simulink model "StraightWithLeadingCar_cs"  (R2016a)
settings: Solver=ode5  SolverMode=SingleTasking  StartTime=0.0  StopTime=40  FixedStep=1/1000  RelTol=1e-3
PreLoadFcn:
  | mbxruntime.callbacks.PreLoadFcn(bdroot);
PostLoadFcn:
  | mbxruntime.callbacks.PostLoadFcn(bdroot);
InitFcn:
  | mbxruntime.callbacks.InitFcn(bdroot);
StartFcn:
  | mbxruntime.callbacks.StartFcn(bdroot);
StopFcn:
  | mbxruntime.callbacks.StopFcn(bdroot);
model workspace (MAT data in the model file):
  mbox_table : struct (value not decoded)
  model_closed = 0
  sim_status = 0
values from neighbouring files (symbols this model uses):
  ACCDuration = 5    [PreScan_Runscript.m]
  V0 = ACCArray(2*ACCCasei-1)    [PreScan_Runscript.m]
  V1 = ACCArray(2*ACCCasei)    [PreScan_Runscript.m]
  VAccuracyIn = 0.8    [PreScan_Runscript.m]
  VDurationIn = 2    [PreScan_Runscript.m]
  VPIDIn = ACCArray(2*ACCCasei-1)    [PreScan_Runscript.m]
  VToleranceIn = 1    [PreScan_Runscript.m]
undefined symbols (not defined in the file or in its folder): ADASID, BMotor1, BMotor2, BrkDelayTime, DControlB, Delay1, Delay2, DiscIntNeverNeededParam, IControlB, JMotor1, JMotor2, mbxruntime, PControlB, PreScanCarSimLoadFcn, ratioGearF, ratioGearR, tabledata, TorqDelayTime, Tstep
undefined symbols (not defined in the file): SteeringColumn, SteeringWheel, WheelL0, WheelL1, WheelR0, WheelR1
libraries: simulink x14, simulink_extras x11, PreScanSimulinkLibrary x9, MyLib x3, Solver_SF x2, PreScanUsefulBlocks x2, pil_lib x1
(part 9 of 12)

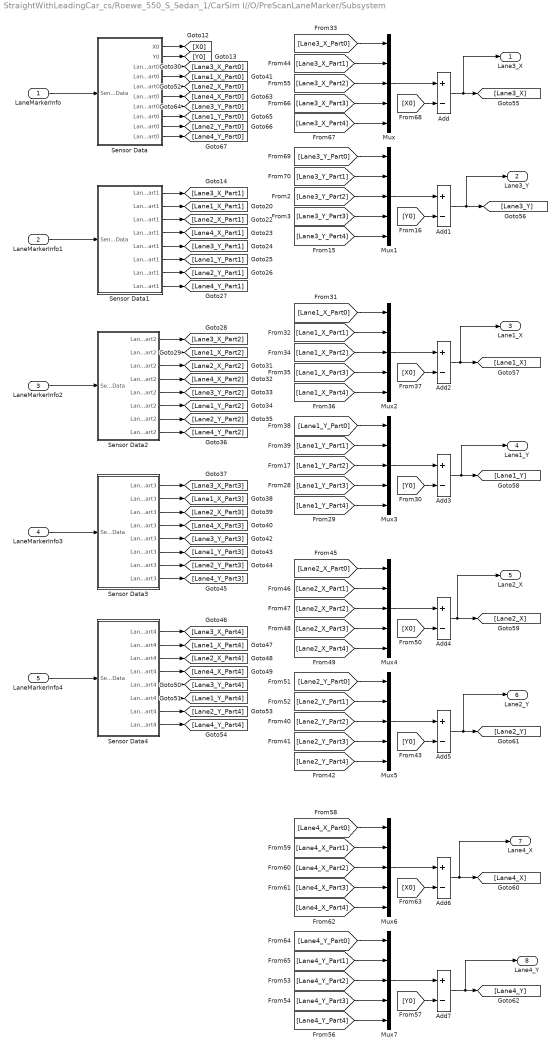
== system StraightWithLeadingCar_cs/Roewe_550_S_Sedan_1/CarSim I//O/PreScanLaneMarker/Subsystem ==
  LaneMarkerInfo : Inport
  LaneMarkerInfo1 : Inport  Port=2
  LaneMarkerInfo2 : Inport  Port=3
  LaneMarkerInfo3 : Inport  Port=4
  LaneMarkerInfo4 : Inport  Port=5
  Add{,1..7} (8 alike) : Sum  Inputs=+-
  Mux{,1..7} (8 alike) : Mux  Inputs=5
  Sensor Data : Subsystem
  Sensor Data1 : Subsystem
  Sensor Data2 : Subsystem
  Sensor Data3 : Subsystem
  Sensor Data4 : Subsystem
  Lane3_X : Outport
  Lane3_Y : Outport  Port=2
  Lane1_X : Outport  Port=3
  Lane1_Y : Outport  Port=4
  Lane2_X : Outport  Port=5
  Lane2_Y : Outport  Port=6
  Lane4_X : Outport  Port=7
  Lane4_Y : Outport  Port=8
  wires:
  [X0] -> Add4/2
  [Lane4_X_Part2] -> Mux6/3
  [Lane2_Y_Part1] -> Mux5/2
  Mux6/1 -> Add6/1
  [Lane4_X_Part0] -> Mux6/1
  [X0] -> Add6/2
  [Lane4_Y_Part4] -> Mux7/5
  Add/1 -> Lane3_X/1, [Lane3_X]
  [Lane4_Y_Part0] -> Mux7/1
  Add3/1 -> Lane1_Y/1, [Lane1_Y]
  [Lane2_Y_Part0] -> Mux5/1
  Mux5/1 -> Add5/1
  Add6/1 -> Lane4_X/1, [Lane4_X]
  [Lane2_Y_Part3] -> Mux5/4
  Mux7/1 -> Add7/1
  Add4/1 -> Lane2_X/1, [Lane2_X]
  Add1/1 -> Lane3_Y/1, [Lane3_Y]
  [Y0] -> Add5/2
  [Lane4_Y_Part1] -> Mux7/2
  [Lane2_Y_Part2] -> Mux5/3
  [Lane4_Y_Part2] -> Mux7/3
  [Lane4_X_Part3] -> Mux6/4
  [Lane4_X_Part4] -> Mux6/5
  [Y0] -> Add7/2
  [Lane4_X_Part1] -> Mux6/2
  Add7/1 -> Lane4_Y/1, [Lane4_Y]
  Add5/1 -> Lane2_Y/1, [Lane2_Y]
  [Lane4_Y_Part3] -> Mux7/4
  [Lane2_Y_Part4] -> Mux5/5
  Sensor Data4/5(Lane3_Y_Part4) -> [Lane3_Y_Part4]
  Sensor Data2/7(Lane2_Y_Part2) -> [Lane2_Y_Part2]
  Sensor Data3/5(Lane3_Y_Part3) -> [Lane3_Y_Part3]
  [Lane3_X_Part3] -> Mux/4
  Sensor Data2/1(Lane3_X_Part2) -> [Lane3_X_Part2]
  Sensor Data3/1(Lane3_X_Part3) -> [Lane3_X_Part3]
  Sensor Data1/8(Lane4_Y_Part1) -> [Lane4_Y_Part1]
  Sensor Data3/3(Lane2_X_Part3) -> [Lane2_X_Part3]
  Sensor Data4/3(Lane2_X_Part4) -> [Lane2_X_Part4]
  Sensor Data2/6(Lane1_Y_Part2) -> [Lane1_Y_Part2]
  Sensor Data1/6(Lane1_Y_Part1) -> [Lane1_Y_Part1]
  Sensor Data3/2(Lane1_X_Part3) -> [Lane1_X_Part3]
  Sensor Data2/3(Lane2_X_Part2) -> [Lane2_X_Part2]
  Sensor Data3/8(Lane4_Y_Part3) -> [Lane4_Y_Part3]
  Sensor Data4/2(Lane1_X_Part4) -> [Lane1_X_Part4]
  Sensor Data3/7(Lane2_Y_Part3) -> [Lane2_Y_Part3]
  Sensor Data4/7(Lane2_Y_Part4) -> [Lane2_Y_Part4]
  Sensor Data3/6(Lane1_Y_Part3) -> [Lane1_Y_Part3]
  [Lane3_X_Part4] -> Mux/5
  [Lane3_X_Part1] -> Mux/2
  Sensor Data4/4(Lane4_X_Part4) -> [Lane4_X_Part4]
  [X0] -> Add/2
  Sensor Data2/2(Lane1_X_Part2) -> [Lane1_X_Part2]
  Sensor Data1/3(Lane2_X_Part1) -> [Lane2_X_Part1]
  Sensor Data4/6(Lane1_Y_Part4) -> [Lane1_Y_Part4]
  [Lane3_X_Part0] -> Mux/1
  Mux/1 -> Add/1
  [Lane3_Y_Part0] -> Mux1/1
  [Lane3_Y_Part2] -> Mux1/3
  [Lane3_Y_Part4] -> Mux1/5
  [Lane3_Y_Part1] -> Mux1/2
  Mux1/1 -> Add1/1
  [Y0] -> Add1/2
  Sensor Data2/8(Lane4_Y_Part2) -> [Lane4_Y_Part2]
  [Lane1_X_Part4] -> Mux2/5
  [Lane1_Y_Part0] -> Mux3/1
  [Lane1_X_Part3] -> Mux2/4
  [Lane1_Y_Part3] -> Mux3/4
  Sensor Data2/5(Lane3_Y_Part2) -> [Lane3_Y_Part2]
  Sensor Data1/7(Lane2_Y_Part1) -> [Lane2_Y_Part1]
  Sensor Data4/1(Lane3_X_Part4) -> [Lane3_X_Part4]
  Sensor Data4/8(Lane4_Y_Part4) -> [Lane4_Y_Part4]
  Sensor Data3/4(Lane4_X_Part3) -> [Lane4_X_Part3]
  Sensor Data2/4(Lane4_X_Part2) -> [Lane4_X_Part2]
  [Lane3_Y_Part3] -> Mux1/4
  Sensor Data1/5(Lane3_Y_Part1) -> [Lane3_Y_Part1]
  [Lane1_X_Part1] -> Mux2/2
  [Lane1_X_Part2] -> Mux2/3
  Mux2/1 -> Add2/1
  [X0] -> Add2/2
  [Lane1_X_Part0] -> Mux2/1
  [Lane1_Y_Part2] -> Mux3/3
  [Lane1_Y_Part4] -> Mux3/5
  [Lane3_X_Part2] -> Mux/3
  [Y0] -> Add3/2
  [Lane2_X_Part0] -> Mux4/1
  [Lane2_X_Part2] -> Mux4/3
  [Lane1_Y_Part1] -> Mux3/2
  Mux3/1 -> Add3/1
  Mux4/1 -> Add4/1
  [Lane2_X_Part3] -> Mux4/4
  [Lane2_X_Part1] -> Mux4/2
  [Lane2_X_Part4] -> Mux4/5
  Sensor Data/2(Y0) -> [Y0]
  Sensor Data/3(Lane3_X_Part0) -> [Lane3_X_Part0]
  Sensor Data/6(Lane4_X_Part0) -> [Lane4_X_Part0]
  Sensor Data/7(Lane3_Y_Part0) -> [Lane3_Y_Part0]
  Sensor Data/1(X0) -> [X0]
  Sensor Data/4(Lane1_X_Part0) -> [Lane1_X_Part0]
  Sensor Data/8(Lane1_Y_Part0) -> [Lane1_Y_Part0]
  Sensor Data/9(Lane2_Y_Part0) -> [Lane2_Y_Part0]
  Sensor Data/10(Lane4_Y_Part0) -> [Lane4_Y_Part0]
  Sensor Data1/1(Lane3_X_Part1) -> [Lane3_X_Part1]
  Sensor Data/5(Lane2_X_Part0) -> [Lane2_X_Part0]
  Sensor Data1/2(Lane1_X_Part1) -> [Lane1_X_Part1]
  Sensor Data1/4(Lane4_X_Part1) -> [Lane4_X_Part1]
  Add2/1 -> Lane1_X/1, [Lane1_X]
  LaneMarkerInfo/1 -> Sensor Data/1(Sensor Data)
  LaneMarkerInfo1/1 -> Sensor Data1/1(Sensor Data)
  LaneMarkerInfo2/1 -> Sensor Data2/1(Sensor Data)
  LaneMarkerInfo3/1 -> Sensor Data3/1(Sensor Data)
  LaneMarkerInfo4/1 -> Sensor Data4/1(Sensor Data)

== system StraightWithLeadingCar_cs/Roewe_550_S_Sedan_1/CarSim_Vehicle/CarSim2PreScanSTATE/Transformation_SprungMassCarSim2PreScan ==
  In1 : Inport
  Demux : Demux  Outputs=3
  Ini z-position VEHICLE wrt GLOBAL axis system [m] : Constant  Value=z0
  Mux : Mux  Inputs=3
  Sum1 : Sum  Inputs=+-
  Out1 : Outport
  wires:
  Mux/1 -> Out1/1
  Ini z-position VEHICLE wrt GLOBAL axis system [m]/1 -> Sum1/2
  Demux/1 -> Mux/1
  Sum1/1 -> Mux/3
  Demux/3 -> Sum1/1
  Demux/2 -> Mux/2
  In1/1 -> Demux/1

== system StraightWithLeadingCar_cs/Roewe_550_S_Sedan_1/CarSim_Vehicle/CarSim2PreScan_BUS/Steering ==
  SteeringWheel_In : Inport
  AvoidDivisionByZero : Subsystem
  Bus Creator4 : BusCreator  Inputs=1
  DefaultValue : Constant  Value=16
  Demux2 : Demux  Outputs=2
  Divide : Product  Inputs=*/
  Switch : Switch  Criteria=u2 ~= 0
  Steering : Outport
  wires:
  AvoidDivisionByZero/1(Out1) -> Divide/2
  Switch/1 -> Bus Creator4/1  "SteeringRatio_[-]"
  DefaultValue/1 -> Switch/3
  Divide/1 -> Switch/1, Switch/2  "Steering_Ration[-]"
  Demux2/2 -> AvoidDivisionByZero/1(In1)  "Axle1ReducedSW"
  Demux2/1 -> Divide/1  "SteeringWheelAngle_[deg]"
  Bus Creator4/1 -> Steering/1  "Steering"
  SteeringWheel_In/1 -> Demux2/1

== system StraightWithLeadingCar_cs/Roewe_550_S_Sedan_1/CarSim_Vehicle/CarSim2PreScan_BUS/Vehicle ==
  v_VehicleCoG[x;y;z][km|h] : Inport
  Bus Creator1 : BusCreator  Inputs=1
  Bus Creator7 : BusCreator  Inputs=1
  Bus Creator8 : BusCreator  Inputs=3
  Demux : Demux  Outputs=3
  Vehicle : Outport
  wires:
  Demux/3 -> Bus Creator8/3  "v_Vehicle[z][km|h]"
  Demux/2 -> Bus Creator8/2  "v_Vehicle[y][km|h]"
  Demux/1 -> Bus Creator8/1  "v_Vehicle[x][km|h]"
  Bus Creator7/1 -> Bus Creator1/1  "Velocities"
  Bus Creator8/1 -> Bus Creator7/1  "Linear"
  Bus Creator1/1 -> Vehicle/1  "Vehicle"
  v_VehicleCoG[x;y;z][km|h]/1 -> Demux/1

== system StraightWithLeadingCar_cs/Roewe_550_S_Sedan_1/CarSim_Vehicle/CarSim2PreScan_BUS/Wheel ==
  SprungMass_Pos_Global[x;y;z][m] : Inport
  SprungMass_Angle_Global[x;y;z][deg] : Inport  Port=2
  CarSim_Pos_Wheel_[FL;FR;RL;RR][x;y;z][m] : Inport  Port=3
  CarSim_Angle_Wheel_[FL;FR;RL;RR][x;y;z][deg;rev;deg] : Inport  Port=4
  Bus Creator3 : BusCreator  Inputs=2
  Bus Creator6 : BusCreator  Inputs=1
  Convert CarSim to PreScan Wheel Position : Subsystem
  Convert CarSim to PreScan Wheel Rotation : Subsystem
  Demux : Demux  Outputs=[3 3 3 3]
  Demux1 : Demux  Outputs=[3 3 3 3]
  Wheel : Outport
  wires:
  SprungMass_Angle_Global[x;y;z][deg]/1 -> Convert CarSim to PreScan Wheel Rotation/5(Angle_Vehicle[x;y;z][deg]), Convert CarSim to PreScan Wheel Position/2(SprungMass_Angle_Global[x;y;z][deg])
  SprungMass_Pos_Global[x;y;z][m]/1 -> Convert CarSim to PreScan Wheel Position/1(SprungMass_Pos_Global[x;y;z][m])
  CarSim_Angle_Wheel_[FL;FR;RL;RR][x;y;z][deg;rev;deg]/1 -> Demux1/1
  Demux1/4 -> Convert CarSim to PreScan Wheel Rotation/4(CarSim_Angle_RR_Wheel_CoorSys_V[deg;rev;deg])  "CarSim_Angle_RR_Wheel_CoorSys_V[deg;rev;deg]"
  Demux1/3 -> Convert CarSim to PreScan Wheel Rotation/3(CarSim_Angle_RL_Wheel_CoorSys_V[deg;rev;deg])  "CarSim_Angle_RL_Wheel_CoorSys_V[deg;rev;deg]"
  Demux1/2 -> Convert CarSim to PreScan Wheel Rotation/2(CarSim_Angle_FR_Wheel_CoorSys_V[deg;rev;deg])  "CarSim_Angle_FR_Wheel_CoorSys_V[deg;rev;deg]"
  Demux1/1 -> Convert CarSim to PreScan Wheel Rotation/1(CarSim_Angle_FL_Wheel_CoorSys_V[deg;rev;deg])  "CarSim_Angle_FL_Wheel_CoorSys_V[deg;rev;deg]"
  CarSim_Pos_Wheel_[FL;FR;RL;RR][x;y;z][m]/1 -> Demux/1
  Demux/4 -> Convert CarSim to PreScan Wheel Position/6(CarSim_Pos_RR_Wheel[x;y;z][m])  "CarSim_Pos_RR_Wheel[x;y;z][m]"
  Demux/3 -> Convert CarSim to PreScan Wheel Position/5(CarSim_Pos_RL_Wheel[x;y;z][m])  "CarSim_Pos_RL_Wheel[x;y;z][m]"
  Demux/2 -> Convert CarSim to PreScan Wheel Position/4(CarSim_Pos_FR_Wheel[x;y;z][m])  "CarSim_Pos_FR_Wheel[x;y;z][m]"
  Demux/1 -> Convert CarSim to PreScan Wheel Position/3(CarSim_Pos_FL_Wheel[x;y;z][m])  "CarSim_Pos_FL_Wheel[x;y;z][m]"
  Bus Creator6/1 -> Wheel/1  "Wheel"
  Bus Creator3/1 -> Bus Creator6/1  "Position"
  Convert CarSim to PreScan Wheel Rotation/1(PreScanWheel_Rot) -> Bus Creator3/2
  Convert CarSim to PreScan Wheel Position/1(PreScanWheel_Pos) -> Bus Creator3/1

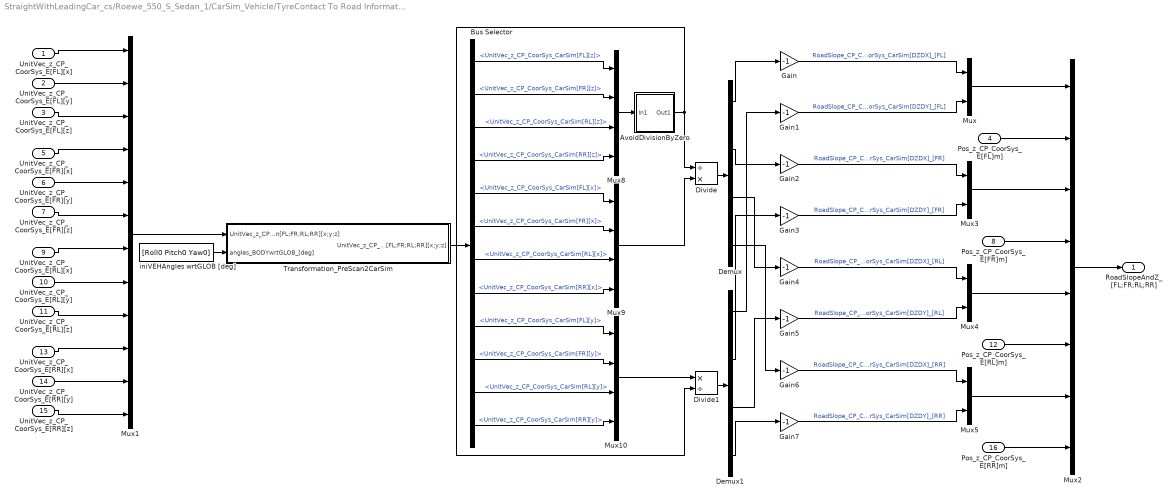
== system StraightWithLeadingCar_cs/Roewe_550_S_Sedan_1/CarSim_Vehicle/TyreContact To Road Information/Contact To Road Information ==
  UnitVec_z_CP_CoorSys_E[FL][x] : Inport
  UnitVec_z_CP_CoorSys_E[FL][y] : Inport  Port=2
  UnitVec_z_CP_CoorSys_E[FL][z] : Inport  Port=3
  " Pos_z_CP_CoorSys_E[FL]m]" : Inport  Port=4
  UnitVec_z_CP_CoorSys_E[FR][x] : Inport  Port=5
  UnitVec_z_CP_CoorSys_E[FR][y] : Inport  Port=6
  UnitVec_z_CP_CoorSys_E[FR][z] : Inport  Port=7
  " Pos_z_CP_CoorSys_E[FR]m]" : Inport  Port=8
  UnitVec_z_CP_CoorSys_E[RL][x] : Inport  Port=9
  UnitVec_z_CP_CoorSys_E[RL][y] : Inport  Port=10
  UnitVec_z_CP_CoorSys_E[RL][z] : Inport  Port=11
  " Pos_z_CP_CoorSys_E[RL]m]" : Inport  Port=12
  UnitVec_z_CP_CoorSys_E[RR][x] : Inport  Port=13
  UnitVec_z_CP_CoorSys_E[RR][y] : Inport  Port=14
  UnitVec_z_CP_CoorSys_E[RR][z] : Inport  Port=15
  " Pos_z_CP_CoorSys_E[RR]m]" : Inport  Port=16
  AvoidDivisionByZero : Subsystem
  Bus Selector : BusSelector  OutputSignals=UnitVec_z_CP_CoorSys_CarSim[FL][x;y;z].UnitVec_z_CP_CoorSys_CarSim[FL][z],UnitVec_z_CP_CoorSys_CarSim[FR][x;y;z].UnitVec_z_CP_CoorSys_CarSim[FR][z],UnitVec_z_CP_CoorSys_CarSim[RL][x;y;z].UnitVec_z_CP_CoorSys_CarSim[RL][z],UnitVec_z_CP_CoorSys_CarSim[RR][x;y;z].UnitVec_z_CP_CoorSys_CarSim[RR][z],UnitVec_z_CP_CoorSys_CarSim[FL][x;y;z].UnitVec_z_CP_CoorSys_CarSim[FL][x],UnitVec_z_CP_CoorSys_CarSim[FR][x;y;z].UnitVec_z_CP_CoorSys_CarSim[FR][x],UnitVec_z_CP_CoorSys_CarSim[RL][x;y;z].UnitVec_z_CP_CoorSys_CarSim[RL][x],UnitVec_z_CP_CoorSys_CarSim[RR][x;y;z].UnitVec_z_CP_CoorSys_CarSim[RR][x],UnitVec_z_CP_CoorSys_CarSim[FL][x;y;z].UnitVec_z_CP_CoorSys_CarSim[FL][y],UnitVec_z_CP_CoorSys_CarSim[FR][x;y;z].UnitVec_z_CP_CoorSys_CarSim[FR][y],UnitVec_z_CP_CoorSys_CarSim[RL][x;y;z].UnitVec_z_CP_CoorSys_CarSim[RL][y],UnitVec_z_CP_CoorSys_CarSim[RR][x;y;z].UnitVec_z_CP_CoorSys_CarSim[RR][y]
  Demux : Demux
  Demux1 : Demux
  Divide : Product  Inputs=/*
  Divide1 : Product  Inputs=*/
  Gain{,1..7} (8 alike) : Gain  Gain=-1
  Mux{,3..5} (4 alike) : Mux  Inputs=2
  Mux1 : Mux  Inputs=12
  Mux10 : Mux
  Mux2 : Mux  Inputs=[2 1 2 1 2 1 2 1]
  Mux8 : Mux
  Mux9 : Mux
  Transformation_PreScan2CarSim : Subsystem
  iniVEHAngles wrtGLOB [deg] : Constant  Value=[Roll0 Pitch0 Yaw0]
  RoadSlopeAndZ_[FL;FR;RL;RR] : Outport
  wires:
  AvoidDivisionByZero/1(Out1) -> Divide1/2, Divide/1
  Demux1/4 -> Gain7/1
  Demux/4 -> Gain6/1
  Demux1/3 -> Gain5/1
  Demux/3 -> Gain4/1
  Demux1/2 -> Gain3/1
  Demux/2 -> Gain2/1
  Demux/1 -> Gain/1
  Demux1/1 -> Gain1/1
  Divide1/1 -> Demux1/1
  Divide/1 -> Demux/1
  Mux10/1 -> Divide1/1
  Mux9/1 -> Divide/2
  Mux8/1 -> AvoidDivisionByZero/1(In1)
  Bus Selector/12 -> Mux10/4  "<UnitVec_z_CP_CoorSys_CarSim[RR][y]>"
  Bus Selector/11 -> Mux10/3  "<UnitVec_z_CP_CoorSys_CarSim[RL][y]>"
  Bus Selector/10 -> Mux10/2  "<UnitVec_z_CP_CoorSys_CarSim[FR][y]>"
  Bus Selector/9 -> Mux10/1  "<UnitVec_z_CP_CoorSys_CarSim[FL][y]>"
  Bus Selector/8 -> Mux9/4  "<UnitVec_z_CP_CoorSys_CarSim[RR][x]>"
  Bus Selector/7 -> Mux9/3  "<UnitVec_z_CP_CoorSys_CarSim[RL][x]>"
  Bus Selector/6 -> Mux9/2  "<UnitVec_z_CP_CoorSys_CarSim[FR][x]>"
  Bus Selector/5 -> Mux9/1  "<UnitVec_z_CP_CoorSys_CarSim[FL][x]>"
  Bus Selector/4 -> Mux8/4  "<UnitVec_z_CP_CoorSys_CarSim[RR][z]>"
  Bus Selector/3 -> Mux8/3  "<UnitVec_z_CP_CoorSys_CarSim[RL][z]>"
  Bus Selector/2 -> Mux8/2  "<UnitVec_z_CP_CoorSys_CarSim[FR][z]>"
  Bus Selector/1 -> Mux8/1  "<UnitVec_z_CP_CoorSys_CarSim[FL][z]>"
  Mux5/1 -> Mux2/7
  Mux4/1 -> Mux2/5
  Mux3/1 -> Mux2/3
  " Pos_z_CP_CoorSys_E[FL]m]"/1 -> Mux2/2
  Mux/1 -> Mux2/1
  Gain/1 -> Mux/1  "RoadSlope_CP_CoorSys_CarSim[DZDX]_[FL]"
  " Pos_z_CP_CoorSys_E[RR]m]"/1 -> Mux2/8
  " Pos_z_CP_CoorSys_E[RL]m]"/1 -> Mux2/6
  " Pos_z_CP_CoorSys_E[FR]m]"/1 -> Mux2/4
  Transformation_PreScan2CarSim/1(UnitVec_z_CP_CoorSys _CarSim[FL;FR;RL;RR][x;y;z]) -> Bus Selector/1
  UnitVec_z_CP_CoorSys_E[RR][z]/1 -> Mux1/12
  UnitVec_z_CP_CoorSys_E[RR][y]/1 -> Mux1/11
  UnitVec_z_CP_CoorSys_E[RR][x]/1 -> Mux1/10
  UnitVec_z_CP_CoorSys_E[RL][z]/1 -> Mux1/9
  UnitVec_z_CP_CoorSys_E[RL][y]/1 -> Mux1/8
  UnitVec_z_CP_CoorSys_E[RL][x]/1 -> Mux1/7
  UnitVec_z_CP_CoorSys_E[FR][z]/1 -> Mux1/6
  UnitVec_z_CP_CoorSys_E[FR][y]/1 -> Mux1/5
  UnitVec_z_CP_CoorSys_E[FR][x]/1 -> Mux1/4
  UnitVec_z_CP_CoorSys_E[FL][z]/1 -> Mux1/3
  UnitVec_z_CP_CoorSys_E[FL][y]/1 -> Mux1/2
  UnitVec_z_CP_CoorSys_E[FL][x]/1 -> Mux1/1
  Mux1/1 -> Transformation_PreScan2CarSim/1(UnitVec_z_CP_CoorSys_PreScan[FL;FR;RL;RR][x;y;z])
  iniVEHAngles wrtGLOB [deg]/1 -> Transformation_PreScan2CarSim/2(angles_BODYwrtGLOB_[deg])
  Mux2/1 -> RoadSlopeAndZ_[FL;FR;RL;RR]/1
  Gain1/1 -> Mux/2  "RoadSlope_CP_CoorSys_CarSim[DZDY]_[FL]"
  Gain2/1 -> Mux3/1  "RoadSlope_CP_CoorSys_CarSim[DZDX]_[FR]"
  Gain3/1 -> Mux3/2  "RoadSlope_CP_CoorSys_CarSim[DZDY]_[FR]"
  Gain4/1 -> Mux4/1  "RoadSlope_CP_CoorSys_CarSim[DZDX]_[RL]"
  Gain5/1 -> Mux4/2  "RoadSlope_CP_CoorSys_CarSim[DZDY]_[RL]"
  Gain6/1 -> Mux5/1  "RoadSlope_CP_CoorSys_CarSim[DZDX]_[RR]"
  Gain7/1 -> Mux5/2  "RoadSlope_CP_CoorSys_CarSim[DZDY]_[RR]"

== system StraightWithLeadingCar_cs/Roewe_550_S_Sedan_1/PreScan_RayCast_Contact_Sensor/Vehicle Local to World/state2FullState ==
  note: AnglesBODY
      | wrtVEH
  note: AnglesVEHICLE
      | wrtGLOB
  note: AnglesBODY
      | wrt GLOB
  note: mode: Dynamics
      | VelVEHICLE
      | wrt VEH
  note: mode: Positioning
      | VelVEHICLE
      | wrt INI
  note: Angles
      | wrtINI
  note: wrt GLOB
  dx,dy,dz [m/s] R,P,Y [rad] : Inport
  ini VEHpos wrt GLOB axis system [m] : Inport  Port=2
  iniBODY Angles wrt VEH axis system [deg] : Inport  Port=3
  iniVEH Angles wrt GLOB axis system [deg] : Inport  Port=4
  Degrees to Radians : simulink_extras/Transformations/Degrees to Radians
  Degrees to Radians1 : simulink_extras/Transformations/Degrees to Radians
  Demux1 : Demux  Outputs=[3 3 3]
  Demux2 : Demux  Outputs=[2 1]
  Demux3 : Demux  Outputs=2
  Mux : Mux  Inputs=[3 3]
  Sum : Sum  Inputs=|++
  Sum1 : Sum
  Sum2 : Sum
  Sum3 : Sum
  Terminator : Terminator
  Transformation_BODY2GLOBAL1 : Subsystem
  limit roll : Subsystem
  mux2 : Mux  Inputs=3
  mux3 : Mux  Inputs=3
  pitch_vehicle : Constant  Value=0
  roll_vehicle : Constant  Value=0
  yaw_body : Constant  Value=0
  State : Outport
  wires:
  Demux1/2 -> Terminator/1
  limit roll/1(RPYcor) -> Mux/2  "AnglesBODY wrt  GLOB"
  Mux/1 -> State/1
  iniVEH Angles wrt GLOB axis system [deg]/1 -> Degrees to Radians/1
  iniBODY Angles wrt VEH axis system [deg]/1 -> Degrees to Radians1/1
  Sum/1 -> limit roll/1(RPY)
  roll_vehicle/1 -> mux3/1  "roll"
  pitch_vehicle/1 -> mux3/2  "pitch"
  mux2/1 -> Sum1/1
  yaw_body/1 -> mux2/3  "yaw"
  mux3/1 -> Sum2/1
  Sum2/1 -> Sum/2
  dx,dy,dz [m/s] R,P,Y [rad]/1 -> Demux1/1
  Demux1/1 -> Transformation_BODY2GLOBAL1/1(POSvector_BODY_[m])
  Sum1/1 -> Sum/1
  Transformation_BODY2GLOBAL1/1(POSvector_GLOBAL_[m]) -> Sum3/1
  Sum3/1 -> Mux/1  "PosVEH wrt  GLOB"
  Demux2/2 -> mux3/3  "yaw"
  Demux2/1 -> Demux3/1
  Demux1/3 -> Demux2/1
  Demux3/1 -> mux2/1  "roll"
  Degrees to Radians1/1 -> Sum1/2
  Degrees to Radians/1 -> Transformation_BODY2GLOBAL1/2(angles_BODYwrtGLOB_[rad]), Sum2/2
  ini VEHpos wrt GLOB axis system [m]/1 -> Sum3/2
  Demux3/2 -> mux2/2  "pitch"

== system StraightWithLeadingCar_cs/Roewe_550_S_Sedan_1/PreScan_RayCast_Contact_Sensor/Wheels = 4/wheelposeFL ==
  vector : Inport  OutDataTypeStr=double  PortDimensions=7
  Bus Creator : BusCreator  Inputs='POSITION','ORIENTATION'  OutDataTypeStr=Bus: PRESCAN_POSEA_DATA  NonVirtualBus=on
  Bus Creator1 : BusCreator  Inputs='X','Y','Z'  OutDataTypeStr=Bus: PRESCAN_XYZ_DATA  NonVirtualBus=on
  Bus Creator3 : BusCreator  Inputs='X','Y','Z','Angle'  OutDataTypeStr=Bus: PRESCAN_AXISANGLE_DATA  NonVirtualBus=on
  Demux : Demux  Outputs=7
  bus : Outport  OutDataTypeStr=Bus: PRESCAN_POSEA_DATA
  wires:
  Bus Creator1/1 -> Bus Creator/1  "POSITION"
  Bus Creator3/1 -> Bus Creator/2  "ORIENTATION"
  Bus Creator/1 -> bus/1
  Demux/1 -> Bus Creator1/1  "X"
  Demux/2 -> Bus Creator1/2  "Y"
  Demux/3 -> Bus Creator1/3  "Z"
  Demux/4 -> Bus Creator3/1  "X"
  Demux/5 -> Bus Creator3/2  "Y"
  Demux/6 -> Bus Creator3/3  "Z"
  Demux/7 -> Bus Creator3/4  "Angle"
  vector/1 -> Demux/1

== system StraightWithLeadingCar_cs/Roewe_550_S_Sedan_1/PreScan_RayCast_Contact_Sensor/Wheels = 4/wheelposeFR ==
  vector : Inport  OutDataTypeStr=double  PortDimensions=7
  Bus Creator : BusCreator  Inputs='POSITION','ORIENTATION'  OutDataTypeStr=Bus: PRESCAN_POSEA_DATA  NonVirtualBus=on
  Bus Creator1 : BusCreator  Inputs='X','Y','Z'  OutDataTypeStr=Bus: PRESCAN_XYZ_DATA  NonVirtualBus=on
  Bus Creator3 : BusCreator  Inputs='X','Y','Z','Angle'  OutDataTypeStr=Bus: PRESCAN_AXISANGLE_DATA  NonVirtualBus=on
  Demux : Demux  Outputs=7
  bus : Outport  OutDataTypeStr=Bus: PRESCAN_POSEA_DATA
  wires:
  Bus Creator1/1 -> Bus Creator/1  "POSITION"
  Bus Creator3/1 -> Bus Creator/2  "ORIENTATION"
  Bus Creator/1 -> bus/1
  Demux/1 -> Bus Creator1/1  "X"
  Demux/2 -> Bus Creator1/2  "Y"
  Demux/3 -> Bus Creator1/3  "Z"
  Demux/4 -> Bus Creator3/1  "X"
  Demux/5 -> Bus Creator3/2  "Y"
  Demux/6 -> Bus Creator3/3  "Z"
  Demux/7 -> Bus Creator3/4  "Angle"
  vector/1 -> Demux/1

== system StraightWithLeadingCar_cs/Roewe_550_S_Sedan_1/PreScan_RayCast_Contact_Sensor/Wheels = 4/wheelposeRL ==
  vector : Inport  OutDataTypeStr=double  PortDimensions=7
  Bus Creator : BusCreator  Inputs='POSITION','ORIENTATION'  OutDataTypeStr=Bus: PRESCAN_POSEA_DATA  NonVirtualBus=on
  Bus Creator1 : BusCreator  Inputs='X','Y','Z'  OutDataTypeStr=Bus: PRESCAN_XYZ_DATA  NonVirtualBus=on
  Bus Creator3 : BusCreator  Inputs='X','Y','Z','Angle'  OutDataTypeStr=Bus: PRESCAN_AXISANGLE_DATA  NonVirtualBus=on
  Demux : Demux  Outputs=7
  bus : Outport  OutDataTypeStr=Bus: PRESCAN_POSEA_DATA
  wires:
  Bus Creator1/1 -> Bus Creator/1  "POSITION"
  Bus Creator3/1 -> Bus Creator/2  "ORIENTATION"
  Bus Creator/1 -> bus/1
  Demux/1 -> Bus Creator1/1  "X"
  Demux/2 -> Bus Creator1/2  "Y"
  Demux/3 -> Bus Creator1/3  "Z"
  Demux/4 -> Bus Creator3/1  "X"
  Demux/5 -> Bus Creator3/2  "Y"
  Demux/6 -> Bus Creator3/3  "Z"
  Demux/7 -> Bus Creator3/4  "Angle"
  vector/1 -> Demux/1

== system StraightWithLeadingCar_cs/Roewe_550_S_Sedan_1/PreScan_RayCast_Contact_Sensor/Wheels = 4/wheelposeRR ==
  vector : Inport  OutDataTypeStr=double  PortDimensions=7
  Bus Creator : BusCreator  Inputs='POSITION','ORIENTATION'  OutDataTypeStr=Bus: PRESCAN_POSEA_DATA  NonVirtualBus=on
  Bus Creator1 : BusCreator  Inputs='X','Y','Z'  OutDataTypeStr=Bus: PRESCAN_XYZ_DATA  NonVirtualBus=on
  Bus Creator3 : BusCreator  Inputs='X','Y','Z','Angle'  OutDataTypeStr=Bus: PRESCAN_AXISANGLE_DATA  NonVirtualBus=on
  Demux : Demux  Outputs=7
  bus : Outport  OutDataTypeStr=Bus: PRESCAN_POSEA_DATA
  wires:
  Bus Creator1/1 -> Bus Creator/1  "POSITION"
  Bus Creator3/1 -> Bus Creator/2  "ORIENTATION"
  Bus Creator/1 -> bus/1
  Demux/1 -> Bus Creator1/1  "X"
  Demux/2 -> Bus Creator1/2  "Y"
  Demux/3 -> Bus Creator1/3  "Z"
  Demux/4 -> Bus Creator3/1  "X"
  Demux/5 -> Bus Creator3/2  "Y"
  Demux/6 -> Bus Creator3/3  "Z"
  Demux/7 -> Bus Creator3/4  "Angle"
  vector/1 -> Demux/1

== system StraightWithLeadingCar_cs/Roewe_550_S_Sedan_1/PreScan_RayCast_Contact_Sensor/Wheels Local to World/conv_RotWheelFL ==
  BryantISO [deg] : Inport
  Fcn10 : Fcn  Expr=cos(u(1))*sin(u(3))+sin(u(1))*sin(u(2))*cos(u(3))
  Fcn11 : Fcn  Expr=sin(u(1))*sin(u(3))-cos(u(1))*sin(u(2))*cos(u(3))
  Fcn12 : Fcn  Expr=-cos(u(2))*sin(u(3))
  Fcn13 : Fcn  Expr=cos(u(1))*cos(u(3))-sin(u(1))*sin(u(2))*sin(u(3))
  Fcn14 : Fcn  Expr=sin(u(1))*cos(u(3))+cos(u(1))*sin(u(2))*sin(u(3))
  Fcn15 : Fcn  Expr=sin(u(2))
  Fcn16 : Fcn  Expr=-sin(u(1))*cos(u(2))
  Fcn17 : Fcn  Expr=cos(u(1))*cos(u(2))
  Fcn9 : Fcn  Expr=cos(u(2))*cos(u(3))
  Mux1 : Mux  Inputs=9
  RotMat2AxisAngle : Subsystem
  deg2rad : Gain  Gain=pi/180
  xyz 2 zxy : Selector  InputPortWidth=3  IndexOptions=Index vector (dialog)  Indices=[3 1 2]  OutputSizes=1
  zxy 2 xyz : Selector  InputPortWidth=4  IndexOptions=Index vector (dialog)  Indices=[2 3 1 4]  OutputSizes=1
  QuaternionVisu [rad] : Outport
  wires:
  Fcn9/1 -> Mux1/1
  Fcn10/1 -> Mux1/2
  Fcn11/1 -> Mux1/3
  Fcn12/1 -> Mux1/4
  Fcn13/1 -> Mux1/5
  Fcn14/1 -> Mux1/6
  Fcn15/1 -> Mux1/7
  Fcn16/1 -> Mux1/8
  Fcn17/1 -> Mux1/9
  Mux1/1 -> RotMat2AxisAngle/1(RotMat_Visu)  "RotationMatrix Visu"
  RotMat2AxisAngle/1(Angles_Visu) -> zxy 2 xyz/1
  BryantISO [deg]/1 -> xyz 2 zxy/1  "BryantAngles rotx roty rotz Visu"
  deg2rad/1 -> Fcn9/1, Fcn10/1, Fcn11/1, Fcn12/1, Fcn13/1, Fcn14/1, Fcn15/1, Fcn16/1, Fcn17/1
  xyz 2 zxy/1 -> deg2rad/1
  zxy 2 xyz/1 -> QuaternionVisu [rad]/1

== system StraightWithLeadingCar_cs/Roewe_550_S_Sedan_1/PreScan_RayCast_Contact_Sensor/Wheels Local to World/conv_RotWheelFR ==
  BryantISO [deg] : Inport
  Fcn10 : Fcn  Expr=cos(u(1))*sin(u(3))+sin(u(1))*sin(u(2))*cos(u(3))
  Fcn11 : Fcn  Expr=sin(u(1))*sin(u(3))-cos(u(1))*sin(u(2))*cos(u(3))
  Fcn12 : Fcn  Expr=-cos(u(2))*sin(u(3))
  Fcn13 : Fcn  Expr=cos(u(1))*cos(u(3))-sin(u(1))*sin(u(2))*sin(u(3))
  Fcn14 : Fcn  Expr=sin(u(1))*cos(u(3))+cos(u(1))*sin(u(2))*sin(u(3))
  Fcn15 : Fcn  Expr=sin(u(2))
  Fcn16 : Fcn  Expr=-sin(u(1))*cos(u(2))
  Fcn17 : Fcn  Expr=cos(u(1))*cos(u(2))
  Fcn9 : Fcn  Expr=cos(u(2))*cos(u(3))
  Mux1 : Mux  Inputs=9
  RotMat2AxisAngle : Subsystem
  deg2rad : Gain  Gain=pi/180
  xyz 2 zxy : Selector  InputPortWidth=3  IndexOptions=Index vector (dialog)  Indices=[3 1 2]  OutputSizes=1
  zxy 2 xyz : Selector  InputPortWidth=4  IndexOptions=Index vector (dialog)  Indices=[2 3 1 4]  OutputSizes=1
  QuaternionVisu [rad] : Outport
  wires:
  Fcn9/1 -> Mux1/1
  Fcn10/1 -> Mux1/2
  Fcn11/1 -> Mux1/3
  Fcn12/1 -> Mux1/4
  Fcn13/1 -> Mux1/5
  Fcn14/1 -> Mux1/6
  Fcn15/1 -> Mux1/7
  Fcn16/1 -> Mux1/8
  Fcn17/1 -> Mux1/9
  Mux1/1 -> RotMat2AxisAngle/1(RotMat_Visu)  "RotationMatrix Visu"
  RotMat2AxisAngle/1(Angles_Visu) -> zxy 2 xyz/1
  BryantISO [deg]/1 -> xyz 2 zxy/1  "BryantAngles rotx roty rotz Visu"
  deg2rad/1 -> Fcn9/1, Fcn10/1, Fcn11/1, Fcn12/1, Fcn13/1, Fcn14/1, Fcn15/1, Fcn16/1, Fcn17/1
  xyz 2 zxy/1 -> deg2rad/1
  zxy 2 xyz/1 -> QuaternionVisu [rad]/1

== system StraightWithLeadingCar_cs/Roewe_550_S_Sedan_1/PreScan_RayCast_Contact_Sensor/Wheels Local to World/conv_RotWheelRL ==
  BryantISO [deg] : Inport
  Fcn10 : Fcn  Expr=cos(u(1))*sin(u(3))+sin(u(1))*sin(u(2))*cos(u(3))
  Fcn11 : Fcn  Expr=sin(u(1))*sin(u(3))-cos(u(1))*sin(u(2))*cos(u(3))
  Fcn12 : Fcn  Expr=-cos(u(2))*sin(u(3))
  Fcn13 : Fcn  Expr=cos(u(1))*cos(u(3))-sin(u(1))*sin(u(2))*sin(u(3))
  Fcn14 : Fcn  Expr=sin(u(1))*cos(u(3))+cos(u(1))*sin(u(2))*sin(u(3))
  Fcn15 : Fcn  Expr=sin(u(2))
  Fcn16 : Fcn  Expr=-sin(u(1))*cos(u(2))
  Fcn17 : Fcn  Expr=cos(u(1))*cos(u(2))
  Fcn9 : Fcn  Expr=cos(u(2))*cos(u(3))
  Mux1 : Mux  Inputs=9
  RotMat2AxisAngle : Subsystem
  deg2rad : Gain  Gain=pi/180
  xyz 2 zxy : Selector  InputPortWidth=3  IndexOptions=Index vector (dialog)  Indices=[3 1 2]  OutputSizes=1
  zxy 2 xyz : Selector  InputPortWidth=4  IndexOptions=Index vector (dialog)  Indices=[2 3 1 4]  OutputSizes=1
  QuaternionVisu [rad] : Outport
  wires:
  Fcn9/1 -> Mux1/1
  Fcn10/1 -> Mux1/2
  Fcn11/1 -> Mux1/3
  Fcn12/1 -> Mux1/4
  Fcn13/1 -> Mux1/5
  Fcn14/1 -> Mux1/6
  Fcn15/1 -> Mux1/7
  Fcn16/1 -> Mux1/8
  Fcn17/1 -> Mux1/9
  Mux1/1 -> RotMat2AxisAngle/1(RotMat_Visu)  "RotationMatrix Visu"
  RotMat2AxisAngle/1(Angles_Visu) -> zxy 2 xyz/1
  BryantISO [deg]/1 -> xyz 2 zxy/1  "BryantAngles rotx roty rotz Visu"
  deg2rad/1 -> Fcn9/1, Fcn10/1, Fcn11/1, Fcn12/1, Fcn13/1, Fcn14/1, Fcn15/1, Fcn16/1, Fcn17/1
  xyz 2 zxy/1 -> deg2rad/1
  zxy 2 xyz/1 -> QuaternionVisu [rad]/1

== system StraightWithLeadingCar_cs/Roewe_550_S_Sedan_1/PreScan_RayCast_Contact_Sensor/Wheels Local to World/conv_RotWheelRR ==
  BryantISO [deg] : Inport
  Fcn10 : Fcn  Expr=cos(u(1))*sin(u(3))+sin(u(1))*sin(u(2))*cos(u(3))
  Fcn11 : Fcn  Expr=sin(u(1))*sin(u(3))-cos(u(1))*sin(u(2))*cos(u(3))
  Fcn12 : Fcn  Expr=-cos(u(2))*sin(u(3))
  Fcn13 : Fcn  Expr=cos(u(1))*cos(u(3))-sin(u(1))*sin(u(2))*sin(u(3))
  Fcn14 : Fcn  Expr=sin(u(1))*cos(u(3))+cos(u(1))*sin(u(2))*sin(u(3))
  Fcn15 : Fcn  Expr=sin(u(2))
  Fcn16 : Fcn  Expr=-sin(u(1))*cos(u(2))
  Fcn17 : Fcn  Expr=cos(u(1))*cos(u(2))
  Fcn9 : Fcn  Expr=cos(u(2))*cos(u(3))
  Mux1 : Mux  Inputs=9
  RotMat2AxisAngle : Subsystem
  deg2rad : Gain  Gain=pi/180
  xyz 2 zxy : Selector  InputPortWidth=3  IndexOptions=Index vector (dialog)  Indices=[3 1 2]  OutputSizes=1
  zxy 2 xyz : Selector  InputPortWidth=4  IndexOptions=Index vector (dialog)  Indices=[2 3 1 4]  OutputSizes=1
  QuaternionVisu [rad] : Outport
  wires:
  Fcn9/1 -> Mux1/1
  Fcn10/1 -> Mux1/2
  Fcn11/1 -> Mux1/3
  Fcn12/1 -> Mux1/4
  Fcn13/1 -> Mux1/5
  Fcn14/1 -> Mux1/6
  Fcn15/1 -> Mux1/7
  Fcn16/1 -> Mux1/8
  Fcn17/1 -> Mux1/9
  Mux1/1 -> RotMat2AxisAngle/1(RotMat_Visu)  "RotationMatrix Visu"
  RotMat2AxisAngle/1(Angles_Visu) -> zxy 2 xyz/1
  BryantISO [deg]/1 -> xyz 2 zxy/1  "BryantAngles rotx roty rotz Visu"
  deg2rad/1 -> Fcn9/1, Fcn10/1, Fcn11/1, Fcn12/1, Fcn13/1, Fcn14/1, Fcn15/1, Fcn16/1, Fcn17/1
  xyz 2 zxy/1 -> deg2rad/1
  zxy 2 xyz/1 -> QuaternionVisu [rad]/1

== system StraightWithLeadingCar_cs/Roewe_550_S_Sedan_1/PreScan_RayCast_Contact_Sensor/Wheels Local to World/conv_TransWheelFL ==
  transISO [m] : Inport
  Gain1 : Gain  Gain=Gain_xISO
  Gain2 : Gain  Gain=Gain_yISO
  Gain3 : Gain  Gain=Gain_zISO
  Mux2 : Mux  Inputs=3
  Sum : Sum  Inputs=|++
  pos_ini_Visu : Subsystem
  transISO2Visu : Subsystem
  transVisu [m] : Outport
  wires:
  transISO2Visu/3(trans_z_Visu) -> Gain3/1
  transISO2Visu/2(trans_y_Visu) -> Gain2/1
  transISO2Visu/1(trans_x_Visu) -> Gain1/1
  transISO [m]/1 -> transISO2Visu/1(transISO)
  Mux2/1 -> Sum/1
  pos_ini_Visu/1(pos_ini_Visu) -> Sum/2
  Sum/1 -> transVisu [m]/1
  Gain1/1 -> Mux2/1
  Gain2/1 -> Mux2/2
  Gain3/1 -> Mux2/3

== system StraightWithLeadingCar_cs/Roewe_550_S_Sedan_1/PreScan_RayCast_Contact_Sensor/Wheels Local to World/conv_TransWheelFR ==
  transISO [m] : Inport
  Gain1 : Gain  Gain=Gain_xISO
  Gain2 : Gain  Gain=Gain_yISO
  Gain3 : Gain  Gain=Gain_zISO
  Mux2 : Mux  Inputs=3
  Sum : Sum  Inputs=|++
  pos_ini_Visu : Subsystem
  transISO2Visu : Subsystem
  transVisu [m] : Outport
  wires:
  transISO2Visu/3(trans_z_Visu) -> Gain3/1
  transISO2Visu/2(trans_y_Visu) -> Gain2/1
  transISO2Visu/1(trans_x_Visu) -> Gain1/1
  transISO [m]/1 -> transISO2Visu/1(transISO)
  Mux2/1 -> Sum/1
  pos_ini_Visu/1(pos_ini_Visu) -> Sum/2
  Sum/1 -> transVisu [m]/1
  Gain1/1 -> Mux2/1
  Gain2/1 -> Mux2/2
  Gain3/1 -> Mux2/3

== system StraightWithLeadingCar_cs/Roewe_550_S_Sedan_1/PreScan_RayCast_Contact_Sensor/Wheels Local to World/conv_TransWheelRL ==
  transISO [m] : Inport
  Gain1 : Gain  Gain=Gain_xISO
  Gain2 : Gain  Gain=Gain_yISO
  Gain3 : Gain  Gain=Gain_zISO
  Mux2 : Mux  Inputs=3
  Sum : Sum  Inputs=|++
  pos_ini_Visu : Subsystem
  transISO2Visu : Subsystem
  transVisu [m] : Outport
  wires:
  transISO2Visu/1(trans_x_Visu) -> Gain1/1
  transISO [m]/1 -> transISO2Visu/1(transISO)
  transISO2Visu/2(trans_y_Visu) -> Gain2/1
  transISO2Visu/3(trans_z_Visu) -> Gain3/1
  Mux2/1 -> Sum/1
  pos_ini_Visu/1(pos_ini_Visu) -> Sum/2
  Sum/1 -> transVisu [m]/1
  Gain1/1 -> Mux2/1
  Gain2/1 -> Mux2/2
  Gain3/1 -> Mux2/3

== system StraightWithLeadingCar_cs/Roewe_550_S_Sedan_1/PreScan_RayCast_Contact_Sensor/Wheels Local to World/conv_TransWheelRR ==
  transISO [m] : Inport
  Gain1 : Gain  Gain=Gain_xISO
  Gain2 : Gain  Gain=Gain_yISO
  Gain3 : Gain  Gain=Gain_zISO
  Mux2 : Mux  Inputs=3
  Sum : Sum  Inputs=|++
  pos_ini_Visu : Subsystem
  transISO2Visu : Subsystem
  transVisu [m] : Outport
  wires:
  transISO2Visu/1(trans_x_Visu) -> Gain1/1
  transISO [m]/1 -> transISO2Visu/1(transISO)
  transISO2Visu/2(trans_y_Visu) -> Gain2/1
  transISO2Visu/3(trans_z_Visu) -> Gain3/1
  Mux2/1 -> Sum/1
  pos_ini_Visu/1(pos_ini_Visu) -> Sum/2
  Sum/1 -> transVisu [m]/1
  Gain1/1 -> Mux2/1
  Gain2/1 -> Mux2/2
  Gain3/1 -> Mux2/3

== system StraightWithLeadingCar_cs/Roewe_550_S_Sedan_1/PreScan_RayCast_Contact_Sensor1/Vehicle Local to World/state2FullState ==
  note: AnglesBODY
      | wrtVEH
  note: AnglesVEHICLE
      | wrtGLOB
  note: AnglesBODY
      | wrt GLOB
  note: mode: Dynamics
      | VelVEHICLE
      | wrt VEH
  note: mode: Positioning
      | VelVEHICLE
      | wrt INI
  note: Angles
      | wrtINI
  note: wrt GLOB
  dx,dy,dz [m/s] R,P,Y [rad] : Inport
  ini VEHpos wrt GLOB axis system [m] : Inport  Port=2
  iniBODY Angles wrt VEH axis system [deg] : Inport  Port=3
  iniVEH Angles wrt GLOB axis system [deg] : Inport  Port=4
  Degrees to Radians : simulink_extras/Transformations/Degrees to Radians
  Degrees to Radians1 : simulink_extras/Transformations/Degrees to Radians
  Demux1 : Demux  Outputs=[3 3 3]
  Demux2 : Demux  Outputs=[2 1]
  Demux3 : Demux  Outputs=2
  Mux : Mux  Inputs=[3 3]
  Sum : Sum  Inputs=|++
  Sum1 : Sum
  Sum2 : Sum
  Sum3 : Sum
  Terminator : Terminator
  Transformation_BODY2GLOBAL1 : Subsystem
  limit roll : Subsystem
  mux2 : Mux  Inputs=3
  mux3 : Mux  Inputs=3
  pitch_vehicle : Constant  Value=0
  roll_vehicle : Constant  Value=0
  yaw_body : Constant  Value=0
  State : Outport
  wires:
  Demux1/2 -> Terminator/1
  limit roll/1(RPYcor) -> Mux/2  "AnglesBODY wrt  GLOB"
  Mux/1 -> State/1
  iniVEH Angles wrt GLOB axis system [deg]/1 -> Degrees to Radians/1
  iniBODY Angles wrt VEH axis system [deg]/1 -> Degrees to Radians1/1
  Sum/1 -> limit roll/1(RPY)
  roll_vehicle/1 -> mux3/1  "roll"
  pitch_vehicle/1 -> mux3/2  "pitch"
  mux2/1 -> Sum1/1
  yaw_body/1 -> mux2/3  "yaw"
  mux3/1 -> Sum2/1
  Sum2/1 -> Sum/2
  dx,dy,dz [m/s] R,P,Y [rad]/1 -> Demux1/1
  Demux1/1 -> Transformation_BODY2GLOBAL1/1(POSvector_BODY_[m])
  Sum1/1 -> Sum/1
  Transformation_BODY2GLOBAL1/1(POSvector_GLOBAL_[m]) -> Sum3/1
  Sum3/1 -> Mux/1  "PosVEH wrt  GLOB"
  Demux2/2 -> mux3/3  "yaw"
  Demux2/1 -> Demux3/1
  Demux1/3 -> Demux2/1
  Demux3/1 -> mux2/1  "roll"
  Degrees to Radians1/1 -> Sum1/2
  Degrees to Radians/1 -> Transformation_BODY2GLOBAL1/2(angles_BODYwrtGLOB_[rad]), Sum2/2
  ini VEHpos wrt GLOB axis system [m]/1 -> Sum3/2
  Demux3/2 -> mux2/2  "pitch"

== system StraightWithLeadingCar_cs/Roewe_550_S_Sedan_1/PreScan_RayCast_Contact_Sensor1/Wheels = 4/wheelposeFL ==
  vector : Inport  OutDataTypeStr=double  PortDimensions=7
  Bus Creator : BusCreator  Inputs='POSITION','ORIENTATION'  OutDataTypeStr=Bus: PRESCAN_POSEA_DATA  NonVirtualBus=on
  Bus Creator1 : BusCreator  Inputs='X','Y','Z'  OutDataTypeStr=Bus: PRESCAN_XYZ_DATA  NonVirtualBus=on
  Bus Creator3 : BusCreator  Inputs='X','Y','Z','Angle'  OutDataTypeStr=Bus: PRESCAN_AXISANGLE_DATA  NonVirtualBus=on
  Demux : Demux  Outputs=7
  bus : Outport  OutDataTypeStr=Bus: PRESCAN_POSEA_DATA
  wires:
  Bus Creator1/1 -> Bus Creator/1  "POSITION"
  Bus Creator3/1 -> Bus Creator/2  "ORIENTATION"
  Bus Creator/1 -> bus/1
  Demux/1 -> Bus Creator1/1  "X"
  Demux/2 -> Bus Creator1/2  "Y"
  Demux/3 -> Bus Creator1/3  "Z"
  Demux/4 -> Bus Creator3/1  "X"
  Demux/5 -> Bus Creator3/2  "Y"
  Demux/6 -> Bus Creator3/3  "Z"
  Demux/7 -> Bus Creator3/4  "Angle"
  vector/1 -> Demux/1

== system StraightWithLeadingCar_cs/Roewe_550_S_Sedan_1/PreScan_RayCast_Contact_Sensor1/Wheels = 4/wheelposeFR ==
  vector : Inport  OutDataTypeStr=double  PortDimensions=7
  Bus Creator : BusCreator  Inputs='POSITION','ORIENTATION'  OutDataTypeStr=Bus: PRESCAN_POSEA_DATA  NonVirtualBus=on
  Bus Creator1 : BusCreator  Inputs='X','Y','Z'  OutDataTypeStr=Bus: PRESCAN_XYZ_DATA  NonVirtualBus=on
  Bus Creator3 : BusCreator  Inputs='X','Y','Z','Angle'  OutDataTypeStr=Bus: PRESCAN_AXISANGLE_DATA  NonVirtualBus=on
  Demux : Demux  Outputs=7
  bus : Outport  OutDataTypeStr=Bus: PRESCAN_POSEA_DATA
  wires:
  Bus Creator1/1 -> Bus Creator/1  "POSITION"
  Bus Creator3/1 -> Bus Creator/2  "ORIENTATION"
  Bus Creator/1 -> bus/1
  Demux/1 -> Bus Creator1/1  "X"
  Demux/2 -> Bus Creator1/2  "Y"
  Demux/3 -> Bus Creator1/3  "Z"
  Demux/4 -> Bus Creator3/1  "X"
  Demux/5 -> Bus Creator3/2  "Y"
  Demux/6 -> Bus Creator3/3  "Z"
  Demux/7 -> Bus Creator3/4  "Angle"
  vector/1 -> Demux/1

== system StraightWithLeadingCar_cs/Roewe_550_S_Sedan_1/PreScan_RayCast_Contact_Sensor1/Wheels = 4/wheelposeRL ==
  vector : Inport  OutDataTypeStr=double  PortDimensions=7
  Bus Creator : BusCreator  Inputs='POSITION','ORIENTATION'  OutDataTypeStr=Bus: PRESCAN_POSEA_DATA  NonVirtualBus=on
  Bus Creator1 : BusCreator  Inputs='X','Y','Z'  OutDataTypeStr=Bus: PRESCAN_XYZ_DATA  NonVirtualBus=on
  Bus Creator3 : BusCreator  Inputs='X','Y','Z','Angle'  OutDataTypeStr=Bus: PRESCAN_AXISANGLE_DATA  NonVirtualBus=on
  Demux : Demux  Outputs=7
  bus : Outport  OutDataTypeStr=Bus: PRESCAN_POSEA_DATA
  wires:
  Bus Creator1/1 -> Bus Creator/1  "POSITION"
  Bus Creator3/1 -> Bus Creator/2  "ORIENTATION"
  Bus Creator/1 -> bus/1
  Demux/1 -> Bus Creator1/1  "X"
  Demux/2 -> Bus Creator1/2  "Y"
  Demux/3 -> Bus Creator1/3  "Z"
  Demux/4 -> Bus Creator3/1  "X"
  Demux/5 -> Bus Creator3/2  "Y"
  Demux/6 -> Bus Creator3/3  "Z"
  Demux/7 -> Bus Creator3/4  "Angle"
  vector/1 -> Demux/1

== system StraightWithLeadingCar_cs/Roewe_550_S_Sedan_1/PreScan_RayCast_Contact_Sensor1/Wheels = 4/wheelposeRR ==
  vector : Inport  OutDataTypeStr=double  PortDimensions=7
  Bus Creator : BusCreator  Inputs='POSITION','ORIENTATION'  OutDataTypeStr=Bus: PRESCAN_POSEA_DATA  NonVirtualBus=on
  Bus Creator1 : BusCreator  Inputs='X','Y','Z'  OutDataTypeStr=Bus: PRESCAN_XYZ_DATA  NonVirtualBus=on
  Bus Creator3 : BusCreator  Inputs='X','Y','Z','Angle'  OutDataTypeStr=Bus: PRESCAN_AXISANGLE_DATA  NonVirtualBus=on
  Demux : Demux  Outputs=7
  bus : Outport  OutDataTypeStr=Bus: PRESCAN_POSEA_DATA
  wires:
  Bus Creator1/1 -> Bus Creator/1  "POSITION"
  Bus Creator3/1 -> Bus Creator/2  "ORIENTATION"
  Bus Creator/1 -> bus/1
  Demux/1 -> Bus Creator1/1  "X"
  Demux/2 -> Bus Creator1/2  "Y"
  Demux/3 -> Bus Creator1/3  "Z"
  Demux/4 -> Bus Creator3/1  "X"
  Demux/5 -> Bus Creator3/2  "Y"
  Demux/6 -> Bus Creator3/3  "Z"
  Demux/7 -> Bus Creator3/4  "Angle"
  vector/1 -> Demux/1

== system StraightWithLeadingCar_cs/Roewe_550_S_Sedan_1/PreScan_RayCast_Contact_Sensor1/Wheels Local to World/conv_RotWheelFL ==
  BryantISO [deg] : Inport
  Fcn10 : Fcn  Expr=cos(u(1))*sin(u(3))+sin(u(1))*sin(u(2))*cos(u(3))
  Fcn11 : Fcn  Expr=sin(u(1))*sin(u(3))-cos(u(1))*sin(u(2))*cos(u(3))
  Fcn12 : Fcn  Expr=-cos(u(2))*sin(u(3))
  Fcn13 : Fcn  Expr=cos(u(1))*cos(u(3))-sin(u(1))*sin(u(2))*sin(u(3))
  Fcn14 : Fcn  Expr=sin(u(1))*cos(u(3))+cos(u(1))*sin(u(2))*sin(u(3))
  Fcn15 : Fcn  Expr=sin(u(2))
  Fcn16 : Fcn  Expr=-sin(u(1))*cos(u(2))
  Fcn17 : Fcn  Expr=cos(u(1))*cos(u(2))
  Fcn9 : Fcn  Expr=cos(u(2))*cos(u(3))
  Mux1 : Mux  Inputs=9
  RotMat2AxisAngle : Subsystem
  deg2rad : Gain  Gain=pi/180
  xyz 2 zxy : Selector  InputPortWidth=3  IndexOptions=Index vector (dialog)  Indices=[3 1 2]  OutputSizes=1
  zxy 2 xyz : Selector  InputPortWidth=4  IndexOptions=Index vector (dialog)  Indices=[2 3 1 4]  OutputSizes=1
  QuaternionVisu [rad] : Outport
  wires:
  Fcn9/1 -> Mux1/1
  Fcn10/1 -> Mux1/2
  Fcn11/1 -> Mux1/3
  Fcn12/1 -> Mux1/4
  Fcn13/1 -> Mux1/5
  Fcn14/1 -> Mux1/6
  Fcn15/1 -> Mux1/7
  Fcn16/1 -> Mux1/8
  Fcn17/1 -> Mux1/9
  Mux1/1 -> RotMat2AxisAngle/1(RotMat_Visu)  "RotationMatrix Visu"
  RotMat2AxisAngle/1(Angles_Visu) -> zxy 2 xyz/1
  BryantISO [deg]/1 -> xyz 2 zxy/1  "BryantAngles rotx roty rotz Visu"
  deg2rad/1 -> Fcn9/1, Fcn10/1, Fcn11/1, Fcn12/1, Fcn13/1, Fcn14/1, Fcn15/1, Fcn16/1, Fcn17/1
  xyz 2 zxy/1 -> deg2rad/1
  zxy 2 xyz/1 -> QuaternionVisu [rad]/1

== system StraightWithLeadingCar_cs/Roewe_550_S_Sedan_1/PreScan_RayCast_Contact_Sensor1/Wheels Local to World/conv_RotWheelFR ==
  BryantISO [deg] : Inport
  Fcn10 : Fcn  Expr=cos(u(1))*sin(u(3))+sin(u(1))*sin(u(2))*cos(u(3))
  Fcn11 : Fcn  Expr=sin(u(1))*sin(u(3))-cos(u(1))*sin(u(2))*cos(u(3))
  Fcn12 : Fcn  Expr=-cos(u(2))*sin(u(3))
  Fcn13 : Fcn  Expr=cos(u(1))*cos(u(3))-sin(u(1))*sin(u(2))*sin(u(3))
  Fcn14 : Fcn  Expr=sin(u(1))*cos(u(3))+cos(u(1))*sin(u(2))*sin(u(3))
  Fcn15 : Fcn  Expr=sin(u(2))
  Fcn16 : Fcn  Expr=-sin(u(1))*cos(u(2))
  Fcn17 : Fcn  Expr=cos(u(1))*cos(u(2))
  Fcn9 : Fcn  Expr=cos(u(2))*cos(u(3))
  Mux1 : Mux  Inputs=9
  RotMat2AxisAngle : Subsystem
  deg2rad : Gain  Gain=pi/180
  xyz 2 zxy : Selector  InputPortWidth=3  IndexOptions=Index vector (dialog)  Indices=[3 1 2]  OutputSizes=1
  zxy 2 xyz : Selector  InputPortWidth=4  IndexOptions=Index vector (dialog)  Indices=[2 3 1 4]  OutputSizes=1
  QuaternionVisu [rad] : Outport
  wires:
  Fcn9/1 -> Mux1/1
  Fcn10/1 -> Mux1/2
  Fcn11/1 -> Mux1/3
  Fcn12/1 -> Mux1/4
  Fcn13/1 -> Mux1/5
  Fcn14/1 -> Mux1/6
  Fcn15/1 -> Mux1/7
  Fcn16/1 -> Mux1/8
  Fcn17/1 -> Mux1/9
  Mux1/1 -> RotMat2AxisAngle/1(RotMat_Visu)  "RotationMatrix Visu"
  RotMat2AxisAngle/1(Angles_Visu) -> zxy 2 xyz/1
  BryantISO [deg]/1 -> xyz 2 zxy/1  "BryantAngles rotx roty rotz Visu"
  deg2rad/1 -> Fcn9/1, Fcn10/1, Fcn11/1, Fcn12/1, Fcn13/1, Fcn14/1, Fcn15/1, Fcn16/1, Fcn17/1
  xyz 2 zxy/1 -> deg2rad/1
  zxy 2 xyz/1 -> QuaternionVisu [rad]/1

== system StraightWithLeadingCar_cs/Roewe_550_S_Sedan_1/PreScan_RayCast_Contact_Sensor1/Wheels Local to World/conv_RotWheelRL ==
  BryantISO [deg] : Inport
  Fcn10 : Fcn  Expr=cos(u(1))*sin(u(3))+sin(u(1))*sin(u(2))*cos(u(3))
  Fcn11 : Fcn  Expr=sin(u(1))*sin(u(3))-cos(u(1))*sin(u(2))*cos(u(3))
  Fcn12 : Fcn  Expr=-cos(u(2))*sin(u(3))
  Fcn13 : Fcn  Expr=cos(u(1))*cos(u(3))-sin(u(1))*sin(u(2))*sin(u(3))
  Fcn14 : Fcn  Expr=sin(u(1))*cos(u(3))+cos(u(1))*sin(u(2))*sin(u(3))
  Fcn15 : Fcn  Expr=sin(u(2))
  Fcn16 : Fcn  Expr=-sin(u(1))*cos(u(2))
  Fcn17 : Fcn  Expr=cos(u(1))*cos(u(2))
  Fcn9 : Fcn  Expr=cos(u(2))*cos(u(3))
  Mux1 : Mux  Inputs=9
  RotMat2AxisAngle : Subsystem
  deg2rad : Gain  Gain=pi/180
  xyz 2 zxy : Selector  InputPortWidth=3  IndexOptions=Index vector (dialog)  Indices=[3 1 2]  OutputSizes=1
  zxy 2 xyz : Selector  InputPortWidth=4  IndexOptions=Index vector (dialog)  Indices=[2 3 1 4]  OutputSizes=1
  QuaternionVisu [rad] : Outport
  wires:
  Fcn9/1 -> Mux1/1
  Fcn10/1 -> Mux1/2
  Fcn11/1 -> Mux1/3
  Fcn12/1 -> Mux1/4
  Fcn13/1 -> Mux1/5
  Fcn14/1 -> Mux1/6
  Fcn15/1 -> Mux1/7
  Fcn16/1 -> Mux1/8
  Fcn17/1 -> Mux1/9
  Mux1/1 -> RotMat2AxisAngle/1(RotMat_Visu)  "RotationMatrix Visu"
  RotMat2AxisAngle/1(Angles_Visu) -> zxy 2 xyz/1
  BryantISO [deg]/1 -> xyz 2 zxy/1  "BryantAngles rotx roty rotz Visu"
  deg2rad/1 -> Fcn9/1, Fcn10/1, Fcn11/1, Fcn12/1, Fcn13/1, Fcn14/1, Fcn15/1, Fcn16/1, Fcn17/1
  xyz 2 zxy/1 -> deg2rad/1
  zxy 2 xyz/1 -> QuaternionVisu [rad]/1

== system StraightWithLeadingCar_cs/Roewe_550_S_Sedan_1/PreScan_RayCast_Contact_Sensor1/Wheels Local to World/conv_RotWheelRR ==
  BryantISO [deg] : Inport
  Fcn10 : Fcn  Expr=cos(u(1))*sin(u(3))+sin(u(1))*sin(u(2))*cos(u(3))
  Fcn11 : Fcn  Expr=sin(u(1))*sin(u(3))-cos(u(1))*sin(u(2))*cos(u(3))
  Fcn12 : Fcn  Expr=-cos(u(2))*sin(u(3))
  Fcn13 : Fcn  Expr=cos(u(1))*cos(u(3))-sin(u(1))*sin(u(2))*sin(u(3))
  Fcn14 : Fcn  Expr=sin(u(1))*cos(u(3))+cos(u(1))*sin(u(2))*sin(u(3))
  Fcn15 : Fcn  Expr=sin(u(2))
  Fcn16 : Fcn  Expr=-sin(u(1))*cos(u(2))
  Fcn17 : Fcn  Expr=cos(u(1))*cos(u(2))
  Fcn9 : Fcn  Expr=cos(u(2))*cos(u(3))
  Mux1 : Mux  Inputs=9
  RotMat2AxisAngle : Subsystem
  deg2rad : Gain  Gain=pi/180
  xyz 2 zxy : Selector  InputPortWidth=3  IndexOptions=Index vector (dialog)  Indices=[3 1 2]  OutputSizes=1
  zxy 2 xyz : Selector  InputPortWidth=4  IndexOptions=Index vector (dialog)  Indices=[2 3 1 4]  OutputSizes=1
  QuaternionVisu [rad] : Outport
  wires:
  Fcn9/1 -> Mux1/1
  Fcn10/1 -> Mux1/2
  Fcn11/1 -> Mux1/3
  Fcn12/1 -> Mux1/4
  Fcn13/1 -> Mux1/5
  Fcn14/1 -> Mux1/6
  Fcn15/1 -> Mux1/7
  Fcn16/1 -> Mux1/8
  Fcn17/1 -> Mux1/9
  Mux1/1 -> RotMat2AxisAngle/1(RotMat_Visu)  "RotationMatrix Visu"
  RotMat2AxisAngle/1(Angles_Visu) -> zxy 2 xyz/1
  BryantISO [deg]/1 -> xyz 2 zxy/1  "BryantAngles rotx roty rotz Visu"
  deg2rad/1 -> Fcn9/1, Fcn10/1, Fcn11/1, Fcn12/1, Fcn13/1, Fcn14/1, Fcn15/1, Fcn16/1, Fcn17/1
  xyz 2 zxy/1 -> deg2rad/1
  zxy 2 xyz/1 -> QuaternionVisu [rad]/1

== system StraightWithLeadingCar_cs/Roewe_550_S_Sedan_1/PreScan_RayCast_Contact_Sensor1/Wheels Local to World/conv_TransWheelFL ==
  transISO [m] : Inport
  Gain1 : Gain  Gain=Gain_xISO
  Gain2 : Gain  Gain=Gain_yISO
  Gain3 : Gain  Gain=Gain_zISO
  Mux2 : Mux  Inputs=3
  Sum : Sum  Inputs=|++
  pos_ini_Visu : Subsystem
  transISO2Visu : Subsystem
  transVisu [m] : Outport
  wires:
  transISO2Visu/3(trans_z_Visu) -> Gain3/1
  transISO2Visu/2(trans_y_Visu) -> Gain2/1
  transISO2Visu/1(trans_x_Visu) -> Gain1/1
  transISO [m]/1 -> transISO2Visu/1(transISO)
  Mux2/1 -> Sum/1
  pos_ini_Visu/1(pos_ini_Visu) -> Sum/2
  Sum/1 -> transVisu [m]/1
  Gain1/1 -> Mux2/1
  Gain2/1 -> Mux2/2
  Gain3/1 -> Mux2/3

== system StraightWithLeadingCar_cs/Roewe_550_S_Sedan_1/PreScan_RayCast_Contact_Sensor1/Wheels Local to World/conv_TransWheelFR ==
  transISO [m] : Inport
  Gain1 : Gain  Gain=Gain_xISO
  Gain2 : Gain  Gain=Gain_yISO
  Gain3 : Gain  Gain=Gain_zISO
  Mux2 : Mux  Inputs=3
  Sum : Sum  Inputs=|++
  pos_ini_Visu : Subsystem
  transISO2Visu : Subsystem
  transVisu [m] : Outport
  wires:
  transISO2Visu/3(trans_z_Visu) -> Gain3/1
  transISO2Visu/2(trans_y_Visu) -> Gain2/1
  transISO2Visu/1(trans_x_Visu) -> Gain1/1
  transISO [m]/1 -> transISO2Visu/1(transISO)
  Mux2/1 -> Sum/1
  pos_ini_Visu/1(pos_ini_Visu) -> Sum/2
  Sum/1 -> transVisu [m]/1
  Gain1/1 -> Mux2/1
  Gain2/1 -> Mux2/2
  Gain3/1 -> Mux2/3

== system StraightWithLeadingCar_cs/Roewe_550_S_Sedan_1/PreScan_RayCast_Contact_Sensor1/Wheels Local to World/conv_TransWheelRL ==
  transISO [m] : Inport
  Gain1 : Gain  Gain=Gain_xISO
  Gain2 : Gain  Gain=Gain_yISO
  Gain3 : Gain  Gain=Gain_zISO
  Mux2 : Mux  Inputs=3
  Sum : Sum  Inputs=|++
  pos_ini_Visu : Subsystem
  transISO2Visu : Subsystem
  transVisu [m] : Outport
  wires:
  transISO2Visu/1(trans_x_Visu) -> Gain1/1
  transISO [m]/1 -> transISO2Visu/1(transISO)
  transISO2Visu/2(trans_y_Visu) -> Gain2/1
  transISO2Visu/3(trans_z_Visu) -> Gain3/1
  Mux2/1 -> Sum/1
  pos_ini_Visu/1(pos_ini_Visu) -> Sum/2
  Sum/1 -> transVisu [m]/1
  Gain1/1 -> Mux2/1
  Gain2/1 -> Mux2/2
  Gain3/1 -> Mux2/3

== system StraightWithLeadingCar_cs/Roewe_550_S_Sedan_1/PreScan_RayCast_Contact_Sensor1/Wheels Local to World/conv_TransWheelRR ==
  transISO [m] : Inport
  Gain1 : Gain  Gain=Gain_xISO
  Gain2 : Gain  Gain=Gain_yISO
  Gain3 : Gain  Gain=Gain_zISO
  Mux2 : Mux  Inputs=3
  Sum : Sum  Inputs=|++
  pos_ini_Visu : Subsystem
  transISO2Visu : Subsystem
  transVisu [m] : Outport
  wires:
  transISO2Visu/1(trans_x_Visu) -> Gain1/1
  transISO [m]/1 -> transISO2Visu/1(transISO)
  transISO2Visu/2(trans_y_Visu) -> Gain2/1
  transISO2Visu/3(trans_z_Visu) -> Gain3/1
  Mux2/1 -> Sum/1
  pos_ini_Visu/1(pos_ini_Visu) -> Sum/2
  Sum/1 -> transVisu [m]/1
  Gain1/1 -> Mux2/1
  Gain2/1 -> Mux2/2
  Gain3/1 -> Mux2/3

== system StraightWithLeadingCar_cs/Roewe_550_S_Sedan_1/SELF_Demux/compas converter/cart2compas ==
  Angle [deg] : Inport
  Constant : Constant  Value=90
  Constant1 : Constant  Value=360
  Gain : Gain  Gain=1/360
  Gain1 : Gain  Gain=360
  Gain2 : Gain  Gain=-1
  Rounding Function : Rounding
  Sum : Sum  Inputs=|-+
  Sum1 : Sum  Inputs=-+|
  Sum2 : Sum  Inputs=++|
  heading [deg] : Outport
  wires:
  Gain/1 -> Rounding Function/1
  Rounding Function/1 -> Gain1/1
  Gain1/1 -> Sum/1
  Angle [deg]/1 -> Sum1/2
  Sum/1 -> Gain2/1
  Sum1/1 -> Gain/1, Sum/2
  Constant/1 -> Sum1/1
  Gain2/1 -> Sum2/2
  Constant1/1 -> Sum2/1
  Sum2/1 -> heading [deg]/1
